simulink model "DDCU_wxt_v02_forA_LabviewV02"  (R2014a)
settings: Solver=FixedStepDiscrete  StartTime=0.0  StopTime=50  FixedStep=0.0005  RelTol=1e-3
InitFcn:
  | Veh_Par_wxt
values from neighbouring files (symbols this model uses):
  ag_thr = 0.4*g    (= 3.924)    [Veh_Par_wxt.m]
  B = 2.25    [Veh_Par_wxt.m]
  bra_pre_em = 12    [Veh_Par_wxt.m]
  bra_pre_gz2 = 12/3    (= 4)    [Veh_Par_wxt.m]
  bra_pre_gz34 = 12/3    (= 4)    [Veh_Par_wxt.m]
  bra_pre_yd = 12/2    (= 6)    [Veh_Par_wxt.m]
  brakepre_dem_data = [0 1 2 3 4 5 6 7 8 9 10 11 12]    [Veh_Par_wxt.m]
  brakeTrq_dem_data = [0 218.198 436.396 654.594 872.792 1090.99 1309.188 1527.386 1745.584 1963.782 2181.98 2400.178 2618.376]    [Veh_Par_wxt.m]
  bratrq_max = 4*2618.376    (= 10473.504)    [Veh_Par_wxt.m]
  eff_tran = 0.75    [Veh_Par_wxt.m]
  G = Mass*g    (= 36297)    [Veh_Par_wxt.m]
  kd1 = 1    [Veh_Par_wxt.m]
  kd2 = 1    [Veh_Par_wxt.m]
  kd3 = 1    [Veh_Par_wxt.m]
  ki1 = 1    [Veh_Par_wxt.m]
  ki2 = 1    [Veh_Par_wxt.m]
  ki3 = 1    [Veh_Par_wxt.m]
  kp1 = 1    [Veh_Par_wxt.m]
  kp2 = 1    [Veh_Par_wxt.m]
  kp3 = 1    [Veh_Par_wxt.m]
  L = 3.12    [Veh_Par_wxt.m]
  premax = 12    [Veh_Par_wxt.m]
  Radius = 0.20    (= 0.2)    [Veh_Par_wxt.m]
  s_opt_yi_add = 0.05    [Veh_Par_wxt.m]
  s_opt_zhuan_add = 0.05    [Veh_Par_wxt.m]
  spd_map_mot = [0 100 200 300 360 400 500 600 700 800 900]*tras_ratio    [Veh_Par_wxt.m]
  spdmax = 900*tras_ratio    (= 5580)    [Veh_Par_wxt.m]
  speed_thr_park = 5/3.6/Radius*30/pi    (= 66.3145596216)    [Veh_Par_wxt.m]
  tras_ratio = 6.2    [Veh_Par_wxt.m]
  trq_map_mot = [1200 1200 1200 1200 1200 1080 864 720 617 540 480]/tras_ratio    [Veh_Par_wxt.m]
  trqmax = 80    [Veh_Par_wxt.m]
  v_thr1_b = 5    [Veh_Par_wxt.m]
  v_thr2_b = 20    [Veh_Par_wxt.m]
  v_thr_park = 5    [Veh_Par_wxt.m]
undefined symbols (not defined in the file or in its folder): DiscIntNeverNeededParam
libraries: simulink x231, ec5744lib x19
(part 1 of 16)
settings Model: Creator=wxt  LastModifiedBy=wxt
settings OptimizationCC: InlineParams=on  InlineInvariantSignals=on  ExpressionFolding=off  RollThreshold=9  StateBitsets=on  DataBitsets=on  UseTempVars=on  ZeroExternalMemoryAtStartup=off  ZeroInternalMemoryAtStartup=off  EfficientFloat2IntCast=on  OptimizeModelRefInitCode=on  LifeSpan=1
settings DebuggingCC: InheritedTsInSrcMsg=none
settings HardwareCC: ProdLargestAtomicInteger=Long  ProdLargestAtomicFloat=Double  ProdIntDivRoundTo=Zero  ProdEndianess=BigEndian  ProdHWDeviceType=Freescale MPC5500
settings RTWCC: SystemTargetFile=ec5744.tlc  MakeCommand=make_rtw optimized_fixed_point=1  GenerateMakefile=off  TemplateMakefile=ec5744_lcc.tmf  PostCodeGenCommand=ec5744_pst_s2(buildInfo)  Description=Target for EC5744  GenerateReport=on  ProcessScript=ec5744_make_rtw_hook  IncludeHyperlinkInReport=on  LaunchReport=on
settings CodeAppCC: IgnoreCustomStorageClasses=off
settings STFCustomTargetCC: ModelReferenceCompliant=off  ConcurrentExecutionCompliant=off  IncludeMdlTerminateFcn=off  GeneratePreprocessorConditionals=Use local settings  CombineOutputUpdateFcns=on  SuppressErrorStatus=on  ERTCustomFileBanners=on  SupportContinuousTime=off  SupportNonInlinedSFcns=off  MATLABClassNameForMDSCustomization=Simulink.SoftwareTarget.ERTCustomization  GRTInterface=off  SystemTargetFile=ec5744.tlc
settings ERTTargetCC: GenerateSampleERTMain=off  ModelReferenceCompliant=off  IncludeMdlTerminateFcn=off  SuppressErrorStatus=on  GenerateASAP2=on  ERTSrcFileBannerTemplate=ec5744_code_template.cgt  ERTHdrFileBannerTemplate=ec5744_code_template.cgt  ERTDataSrcFileTemplate=ec5744_code_template.cgt  ERTDataHdrFileTemplate=ec5744_code_template.cgt  ERTCustomFileTemplate=ec5744_file_process.tlc

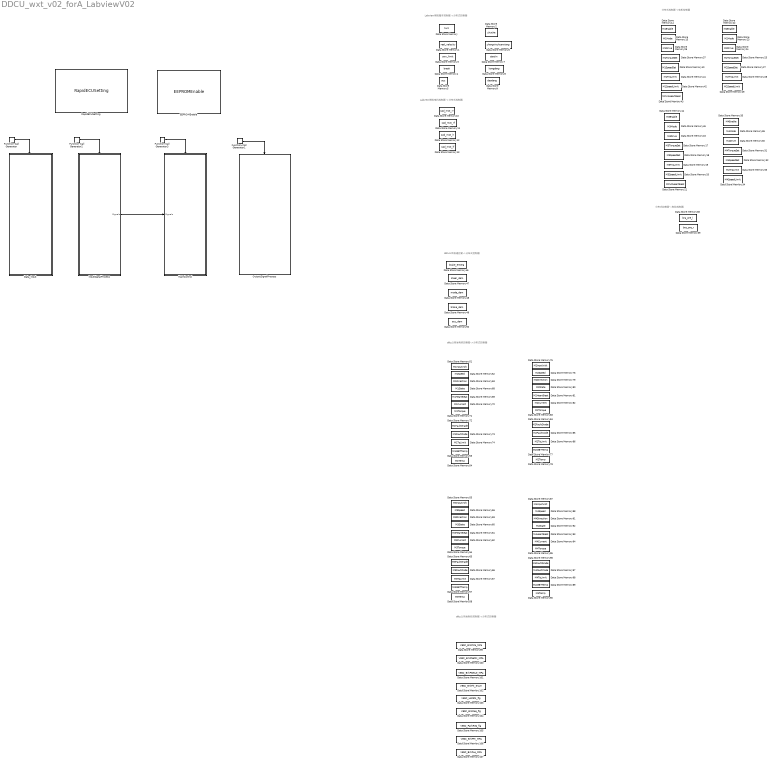
== system DDCU_wxt_v02_forA_LabviewV02 ==
  note: ddcu1转发制动控制器->分布式控制器
  note: ddcu1转发电机控制器->分布式控制器
  note: ddcu1转发遥控箱->分布式控制器
  note: Labview模拟电机控制器->分布式控制器
  note: Labview模拟整车控制器->分布式控制器
  note: 分布式控制器->制动控制器
  note: 分布式控制器->电机控制器
  Data Store Memory : DataStoreMemory  DataStoreName=turn  ReadBeforeWriteMsg=warning  WriteAfterWriteMsg=warning  WriteAfterReadMsg=warning
  Data Store Memory1 : DataStoreMemory  DataStoreName=real_velocity  ReadBeforeWriteMsg=warning  WriteAfterWriteMsg=warning  WriteAfterReadMsg=warning
  Data Store Memory10 : DataStoreMemory  DataStoreName=spd_mot_rr  ReadBeforeWriteMsg=warning  WriteAfterWriteMsg=warning  WriteAfterReadMsg=warning
  Data Store Memory100 : DataStoreMemory  DataStoreName=VESC_BrkPSetRi_MPa  ReadBeforeWriteMsg=warning  WriteAfterWriteMsg=warning  WriteAfterReadMsg=warning
  Data Store Memory101 : DataStoreMemory  DataStoreName=VESC_BrkPSetLe_MPa  ReadBeforeWriteMsg=warning  WriteAfterWriteMsg=warning  WriteAfterReadMsg=warning
  Data Store Memory102 : DataStoreMemory  DataStoreName=VESC_BrkFlt_enum  ReadBeforeWriteMsg=warning  WriteAfterWriteMsg=warning  WriteAfterReadMsg=warning
  Data Store Memory103 : DataStoreMemory  DataStoreName=VESC_HotSts_flg  ReadBeforeWriteMsg=warning  WriteAfterWriteMsg=warning  WriteAfterReadMsg=warning
  Data Store Memory104 : DataStoreMemory  DataStoreName=VESC_BrkReq_flg  ReadBeforeWriteMsg=warning  WriteAfterWriteMsg=warning  WriteAfterReadMsg=warning
  Data Store Memory105 : DataStoreMemory  DataStoreName=VESC_ParkReq_flg  ReadBeforeWriteMsg=warning  WriteAfterWriteMsg=warning  WriteAfterReadMsg=warning
  Data Store Memory106 : DataStoreMemory  DataStoreName=VESC_BrkPRi_MPa  ReadBeforeWriteMsg=warning  WriteAfterWriteMsg=warning  WriteAfterReadMsg=warning
  Data Store Memory107 : DataStoreMemory  DataStoreName=VESC_BrkPLe_MPa  ReadBeforeWriteMsg=warning  WriteAfterWriteMsg=warning  WriteAfterReadMsg=warning
  Data Store Memory11 : DataStoreMemory  DataStoreName=spd_mot_rf  ReadBeforeWriteMsg=warning  WriteAfterWriteMsg=warning  WriteAfterReadMsg=warning
  Data Store Memory12 : DataStoreMemory  DataStoreName=spd_mot_lr  ReadBeforeWriteMsg=warning  WriteAfterWriteMsg=warning  WriteAfterReadMsg=warning
  Data Store Memory13 : DataStoreMemory  DataStoreName=spd_mot_lf  ReadBeforeWriteMsg=warning  WriteAfterWriteMsg=warning  WriteAfterReadMsg=warning
  Data Store Memory14 : DataStoreMemory  DataStoreName=M1Enable  ReadBeforeWriteMsg=warning  WriteAfterWriteMsg=warning  WriteAfterReadMsg=warning
  Data Store Memory15 : DataStoreMemory  DataStoreName=M1Mode  ReadBeforeWriteMsg=warning  WriteAfterWriteMsg=warning  WriteAfterReadMsg=warning
  Data Store Memory16 : DataStoreMemory  DataStoreName=M3Drive  ReadBeforeWriteMsg=warning  WriteAfterWriteMsg=warning  WriteAfterReadMsg=warning
  Data Store Memory17 : DataStoreMemory  DataStoreName=M3TorqueSet  ReadBeforeWriteMsg=warning  WriteAfterWriteMsg=warning  WriteAfterReadMsg=warning
  Data Store Memory18 : DataStoreMemory  DataStoreName=M3SpeedSet  ReadBeforeWriteMsg=warning  WriteAfterWriteMsg=warning  WriteAfterReadMsg=warning
  Data Store Memory19 : DataStoreMemory  DataStoreName=M3TrqLimit  ReadBeforeWriteMsg=warning  WriteAfterWriteMsg=warning  WriteAfterReadMsg=warning
  Data Store Memory2 : DataStoreMemory  DataStoreName=zhuche  ReadBeforeWriteMsg=warning  WriteAfterWriteMsg=warning  WriteAfterReadMsg=warning
  Data Store Memory20 : DataStoreMemory  DataStoreName=M3SpeedLimit  ReadBeforeWriteMsg=warning  WriteAfterWriteMsg=warning  WriteAfterReadMsg=warning
  Data Store Memory21 : DataStoreMemory  DataStoreName=MCU2HeartBeat  ReadBeforeWriteMsg=warning  WriteAfterWriteMsg=warning  WriteAfterReadMsg=warning
  Data Store Memory22 : DataStoreMemory  DataStoreName=M2Enable  ReadBeforeWriteMsg=warning  WriteAfterWriteMsg=warning  WriteAfterReadMsg=warning
  Data Store Memory23 : DataStoreMemory  DataStoreName=M2Mode  ReadBeforeWriteMsg=warning  WriteAfterWriteMsg=warning  WriteAfterReadMsg=warning
  Data Store Memory24 : DataStoreMemory  DataStoreName=M2Drive  ReadBeforeWriteMsg=warning  WriteAfterWriteMsg=warning  WriteAfterReadMsg=warning
  Data Store Memory25 : DataStoreMemory  DataStoreName=M2TorqueSet  ReadBeforeWriteMsg=warning  WriteAfterWriteMsg=warning  WriteAfterReadMsg=warning
  Data Store Memory26 : DataStoreMemory  DataStoreName=M1Drive  ReadBeforeWriteMsg=warning  WriteAfterWriteMsg=warning  WriteAfterReadMsg=warning
  Data Store Memory27 : DataStoreMemory  DataStoreName=M2SpeedSet  ReadBeforeWriteMsg=warning  WriteAfterWriteMsg=warning  WriteAfterReadMsg=warning
  Data Store Memory28 : DataStoreMemory  DataStoreName=M2TrqLimit  ReadBeforeWriteMsg=warning  WriteAfterWriteMsg=warning  WriteAfterReadMsg=warning
  Data Store Memory29 : DataStoreMemory  DataStoreName=M2SpeedLimit  ReadBeforeWriteMsg=warning  WriteAfterWriteMsg=warning  WriteAfterReadMsg=warning
  Data Store Memory3 : DataStoreMemory  DataStoreName=pwr_limit  ReadBeforeWriteMsg=warning  WriteAfterWriteMsg=warning  WriteAfterReadMsg=warning
  Data Store Memory30 : DataStoreMemory  DataStoreName=M4Drive  ReadBeforeWriteMsg=warning  WriteAfterWriteMsg=warning  WriteAfterReadMsg=warning
  Data Store Memory31 : DataStoreMemory  DataStoreName=M4TorqueSet  ReadBeforeWriteMsg=warning  WriteAfterWriteMsg=warning  WriteAfterReadMsg=warning
  Data Store Memory32 : DataStoreMemory  DataStoreName=M4SpeedSet  ReadBeforeWriteMsg=warning  WriteAfterWriteMsg=warning  WriteAfterReadMsg=warning
  Data Store Memory33 : DataStoreMemory  DataStoreName=M4TrqLimit  ReadBeforeWriteMsg=warning  WriteAfterWriteMsg=warning  WriteAfterReadMsg=warning
  Data Store Memory34 : DataStoreMemory  DataStoreName=M4SpeedLimit  ReadBeforeWriteMsg=warning  WriteAfterWriteMsg=warning  WriteAfterReadMsg=warning
  Data Store Memory35 : DataStoreMemory  DataStoreName=M4Enable  ReadBeforeWriteMsg=warning  WriteAfterWriteMsg=warning  WriteAfterReadMsg=warning
  Data Store Memory36 : DataStoreMemory  DataStoreName=M4Mode  ReadBeforeWriteMsg=warning  WriteAfterWriteMsg=warning  WriteAfterReadMsg=warning
  Data Store Memory37 : DataStoreMemory  DataStoreName=M1TorqueSet  ReadBeforeWriteMsg=warning  WriteAfterWriteMsg=warning  WriteAfterReadMsg=warning
  Data Store Memory38 : DataStoreMemory  DataStoreName=bra_pre_l  ReadBeforeWriteMsg=warning  WriteAfterWriteMsg=warning  WriteAfterReadMsg=warning
  Data Store Memory39 : DataStoreMemory  DataStoreName=bra_pre_r  ReadBeforeWriteMsg=warning  WriteAfterWriteMsg=warning  WriteAfterReadMsg=warning
  Data Store Memory4 : DataStoreMemory  DataStoreName=break  ReadBeforeWriteMsg=warning  WriteAfterWriteMsg=warning  WriteAfterReadMsg=warning
  Data Store Memory40 : DataStoreMemory  DataStoreName=M1SpeedSet  ReadBeforeWriteMsg=warning  WriteAfterWriteMsg=warning  WriteAfterReadMsg=warning
  Data Store Memory41 : DataStoreMemory  DataStoreName=M1TrqLimit  ReadBeforeWriteMsg=warning  WriteAfterWriteMsg=warning  WriteAfterReadMsg=warning
  Data Store Memory42 : DataStoreMemory  DataStoreName=M1SpeedLimit  ReadBeforeWriteMsg=warning  WriteAfterWriteMsg=warning  WriteAfterReadMsg=warning
  Data Store Memory43 : DataStoreMemory  DataStoreName=MCU1HeartBeat  ReadBeforeWriteMsg=warning  WriteAfterWriteMsg=warning  WriteAfterReadMsg=warning
  Data Store Memory44 : DataStoreMemory  DataStoreName=M3Enable  ReadBeforeWriteMsg=warning  WriteAfterWriteMsg=warning  WriteAfterReadMsg=warning
  Data Store Memory45 : DataStoreMemory  DataStoreName=M3Mode  ReadBeforeWriteMsg=warning  WriteAfterWriteMsg=warning  WriteAfterReadMsg=warning
  Data Store Memory46 : DataStoreMemory  DataStoreName=brake_emerg  ReadBeforeWriteMsg=warning  WriteAfterWriteMsg=warning  WriteAfterReadMsg=warning
  Data Store Memory47 : DataStoreMemory  DataStoreName=steer_dem  ReadBeforeWriteMsg=warning  WriteAfterWriteMsg=warning  WriteAfterReadMsg=warning
  Data Store Memory48 : DataStoreMemory  DataStoreName=mode_dem  ReadBeforeWriteMsg=warning  WriteAfterWriteMsg=warning  WriteAfterReadMsg=warning
  Data Store Memory49 : DataStoreMemory  DataStoreName=brake_dem  ReadBeforeWriteMsg=warning  WriteAfterWriteMsg=warning  WriteAfterReadMsg=warning
  Data Store Memory5 : DataStoreMemory  DataStoreName=acc  ReadBeforeWriteMsg=warning  WriteAfterWriteMsg=warning  WriteAfterReadMsg=warning
  Data Store Memory50 : DataStoreMemory  DataStoreName=acc_dem  ReadBeforeWriteMsg=warning  WriteAfterWriteMsg=warning  WriteAfterReadMsg=warning
  Data Store Memory51 : DataStoreMemory  DataStoreName=M1InputVolt  ReadBeforeWriteMsg=warning  WriteAfterWriteMsg=warning  WriteAfterReadMsg=warning
  Data Store Memory52 : DataStoreMemory  DataStoreName=M1Speed  ReadBeforeWriteMsg=warning  WriteAfterWriteMsg=warning  WriteAfterReadMsg=warning
  Data Store Memory53 : DataStoreMemory  DataStoreName=M1IGBTTemp  ReadBeforeWriteMsg=warning  WriteAfterWriteMsg=warning  WriteAfterReadMsg=warning
  Data Store Memory54 : DataStoreMemory  DataStoreName=M1Temp  ReadBeforeWriteMsg=warning  WriteAfterWriteMsg=warning  WriteAfterReadMsg=warning
  Data Store Memory55 : DataStoreMemory  DataStoreName=M3InputVolt  ReadBeforeWriteMsg=warning  WriteAfterWriteMsg=warning  WriteAfterReadMsg=warning
  Data Store Memory56 : DataStoreMemory  DataStoreName=M3Speed  ReadBeforeWriteMsg=warning  WriteAfterWriteMsg=warning  WriteAfterReadMsg=warning
  Data Store Memory57 : DataStoreMemory  DataStoreName=M3IGBTTemp  ReadBeforeWriteMsg=warning  WriteAfterWriteMsg=warning  WriteAfterReadMsg=warning
  Data Store Memory58 : DataStoreMemory  DataStoreName=M3Temp  ReadBeforeWriteMsg=warning  WriteAfterWriteMsg=warning  WriteAfterReadMsg=warning
  Data Store Memory59 : DataStoreMemory  DataStoreName=M3Direction  ReadBeforeWriteMsg=warning  WriteAfterWriteMsg=warning  WriteAfterReadMsg=warning
  Data Store Memory6 : DataStoreMemory  DataStoreName=zhongxinzhuanxiang  ReadBeforeWriteMsg=warning  WriteAfterWriteMsg=warning  WriteAfterReadMsg=warning
  Data Store Memory60 : DataStoreMemory  DataStoreName=M3State  ReadBeforeWriteMsg=warning  WriteAfterWriteMsg=warning  WriteAfterReadMsg=warning
  Data Store Memory61 : DataStoreMemory  DataStoreName=M3HeartBeat  ReadBeforeWriteMsg=warning  WriteAfterWriteMsg=warning  WriteAfterReadMsg=warning
  Data Store Memory62 : DataStoreMemory  DataStoreName=M3Current  ReadBeforeWriteMsg=warning  WriteAfterWriteMsg=warning  WriteAfterReadMsg=warning
  Data Store Memory63 : DataStoreMemory  DataStoreName=M1Direction  ReadBeforeWriteMsg=warning  WriteAfterWriteMsg=warning  WriteAfterReadMsg=warning
  Data Store Memory64 : DataStoreMemory  DataStoreName=M3Torque  ReadBeforeWriteMsg=warning  WriteAfterWriteMsg=warning  WriteAfterReadMsg=warning
  Data Store Memory65 : DataStoreMemory  DataStoreName=M3FaultGrade  ReadBeforeWriteMsg=warning  WriteAfterWriteMsg=warning  WriteAfterReadMsg=warning
  Data Store Memory66 : DataStoreMemory  DataStoreName=M3FaultCode  ReadBeforeWriteMsg=warning  WriteAfterWriteMsg=warning  WriteAfterReadMsg=warning
  Data Store Memory67 : DataStoreMemory  DataStoreName=M3TqLimit  ReadBeforeWriteMsg=warning  WriteAfterWriteMsg=warning  WriteAfterReadMsg=warning
  Data Store Memory68 : DataStoreMemory  DataStoreName=M1State  ReadBeforeWriteMsg=warning  WriteAfterWriteMsg=warning  WriteAfterReadMsg=warning
  Data Store Memory69 : DataStoreMemory  DataStoreName=M1HeartBeat  ReadBeforeWriteMsg=warning  WriteAfterWriteMsg=warning  WriteAfterReadMsg=warning
  Data Store Memory7 : DataStoreMemory  DataStoreName=qianjin  ReadBeforeWriteMsg=warning  WriteAfterWriteMsg=warning  WriteAfterReadMsg=warning
  Data Store Memory70 : DataStoreMemory  DataStoreName=M1Current  ReadBeforeWriteMsg=warning  WriteAfterWriteMsg=warning  WriteAfterReadMsg=warning
  Data Store Memory71 : DataStoreMemory  DataStoreName=M1Torque  ReadBeforeWriteMsg=warning  WriteAfterWriteMsg=warning  WriteAfterReadMsg=warning
  Data Store Memory72 : DataStoreMemory  DataStoreName=M1FaultGrade  ReadBeforeWriteMsg=warning  WriteAfterWriteMsg=warning  WriteAfterReadMsg=warning
  Data Store Memory73 : DataStoreMemory  DataStoreName=M1FaultCode  ReadBeforeWriteMsg=warning  WriteAfterWriteMsg=warning  WriteAfterReadMsg=warning
  Data Store Memory74 : DataStoreMemory  DataStoreName=M1TqLimit  ReadBeforeWriteMsg=warning  WriteAfterWriteMsg=warning  WriteAfterReadMsg=warning
  Data Store Memory75 : DataStoreMemory  DataStoreName=M2InputVolt  ReadBeforeWriteMsg=warning  WriteAfterWriteMsg=warning  WriteAfterReadMsg=warning
  Data Store Memory76 : DataStoreMemory  DataStoreName=M2Speed  ReadBeforeWriteMsg=warning  WriteAfterWriteMsg=warning  WriteAfterReadMsg=warning
  Data Store Memory77 : DataStoreMemory  DataStoreName=M2IGBTTemp  ReadBeforeWriteMsg=warning  WriteAfterWriteMsg=warning  WriteAfterReadMsg=warning
  Data Store Memory78 : DataStoreMemory  DataStoreName=M2Temp  ReadBeforeWriteMsg=warning  WriteAfterWriteMsg=warning  WriteAfterReadMsg=warning
  Data Store Memory79 : DataStoreMemory  DataStoreName=M2Direction  ReadBeforeWriteMsg=warning  WriteAfterWriteMsg=warning  WriteAfterReadMsg=warning
  Data Store Memory8 : DataStoreMemory  DataStoreName=kongdang  ReadBeforeWriteMsg=warning  WriteAfterWriteMsg=warning  WriteAfterReadMsg=warning
  Data Store Memory80 : DataStoreMemory  DataStoreName=M2State  ReadBeforeWriteMsg=warning  WriteAfterWriteMsg=warning  WriteAfterReadMsg=warning
  Data Store Memory81 : DataStoreMemory  DataStoreName=M2HeartBeat  ReadBeforeWriteMsg=warning  WriteAfterWriteMsg=warning  WriteAfterReadMsg=warning
  Data Store Memory82 : DataStoreMemory  DataStoreName=M2Current  ReadBeforeWriteMsg=warning  WriteAfterWriteMsg=warning  WriteAfterReadMsg=warning
  Data Store Memory83 : DataStoreMemory  DataStoreName=M2Torque  ReadBeforeWriteMsg=warning  WriteAfterWriteMsg=warning  WriteAfterReadMsg=warning
  Data Store Memory84 : DataStoreMemory  DataStoreName=M2FaultGrade  ReadBeforeWriteMsg=warning  WriteAfterWriteMsg=warning  WriteAfterReadMsg=warning
  Data Store Memory85 : DataStoreMemory  DataStoreName=M2FaultCode  ReadBeforeWriteMsg=warning  WriteAfterWriteMsg=warning  WriteAfterReadMsg=warning
  Data Store Memory86 : DataStoreMemory  DataStoreName=M2TqLimit  ReadBeforeWriteMsg=warning  WriteAfterWriteMsg=warning  WriteAfterReadMsg=warning
  Data Store Memory87 : DataStoreMemory  DataStoreName=M4InputVolt  ReadBeforeWriteMsg=warning  WriteAfterWriteMsg=warning  WriteAfterReadMsg=warning
  Data Store Memory88 : DataStoreMemory  DataStoreName=M4Speed  ReadBeforeWriteMsg=warning  WriteAfterWriteMsg=warning  WriteAfterReadMsg=warning
  Data Store Memory89 : DataStoreMemory  DataStoreName=M4IGBTTemp  ReadBeforeWriteMsg=warning  WriteAfterWriteMsg=warning  WriteAfterReadMsg=warning
  Data Store Memory9 : DataStoreMemory  DataStoreName=daodang  ReadBeforeWriteMsg=warning  WriteAfterWriteMsg=warning  WriteAfterReadMsg=warning
  Data Store Memory90 : DataStoreMemory  DataStoreName=M4Temp  ReadBeforeWriteMsg=warning  WriteAfterWriteMsg=warning  WriteAfterReadMsg=warning
  Data Store Memory91 : DataStoreMemory  DataStoreName=M4Direction  ReadBeforeWriteMsg=warning  WriteAfterWriteMsg=warning  WriteAfterReadMsg=warning
  Data Store Memory92 : DataStoreMemory  DataStoreName=M4State  ReadBeforeWriteMsg=warning  WriteAfterWriteMsg=warning  WriteAfterReadMsg=warning
  Data Store Memory93 : DataStoreMemory  DataStoreName=M4HeartBeat  ReadBeforeWriteMsg=warning  WriteAfterWriteMsg=warning  WriteAfterReadMsg=warning
  Data Store Memory94 : DataStoreMemory  DataStoreName=M4Current  ReadBeforeWriteMsg=warning  WriteAfterWriteMsg=warning  WriteAfterReadMsg=warning
  Data Store Memory95 : DataStoreMemory  DataStoreName=M4Torque  ReadBeforeWriteMsg=warning  WriteAfterWriteMsg=warning  WriteAfterReadMsg=warning
  Data Store Memory96 : DataStoreMemory  DataStoreName=M4FaultGrade  ReadBeforeWriteMsg=warning  WriteAfterWriteMsg=warning  WriteAfterReadMsg=warning
  Data Store Memory97 : DataStoreMemory  DataStoreName=M4FaultCode  ReadBeforeWriteMsg=warning  WriteAfterWriteMsg=warning  WriteAfterReadMsg=warning
  Data Store Memory98 : DataStoreMemory  DataStoreName=M4TqLimit  ReadBeforeWriteMsg=warning  WriteAfterWriteMsg=warning  WriteAfterReadMsg=warning
  Data Store Memory99 : DataStoreMemory  DataStoreName=VESC_BrkPMa_MPa  ReadBeforeWriteMsg=warning  WriteAfterWriteMsg=warning  WriteAfterReadMsg=warning
  Data_Input : Subsystem  TreatAsAtomicUnit=on
  EEPROMEnable : ec5744lib/RapidECU_U3/09MemoryManagement/EEPROMEnable  eepromenable=on
  Function-Call Generator{,1..3} (4 alike) : simulink/Ports & Subsystems/Function-Call Generator  sample_time=0.05  numberOfIterations=1
  InputSignalProcess : Subsystem
  MainControl : Subsystem
  OutputSignalProcess : Subsystem  TreatAsAtomicUnit=on
  RapidECUSetting : ec5744lib/RapidECU_U3/RapidECUSetting
      link override CAN: apdf=4  bpdf=4  cpdf=4  acmt=Extended(29-bit ID)  bcmt=Extended(29-bit ID)
      link override LIN: abrt=19200
  wires:
  Function-Call Generator/1 -> Data_Input/Trigger
  Function-Call Generator1/1 -> OutputSignalProcess/Trigger
  Function-Call Generator2/1 -> InputSignalProcess/Trigger
  InputSignalProcess/1(Signals) -> MainControl/1(Signals)
  Function-Call Generator3/1 -> MainControl/Trigger

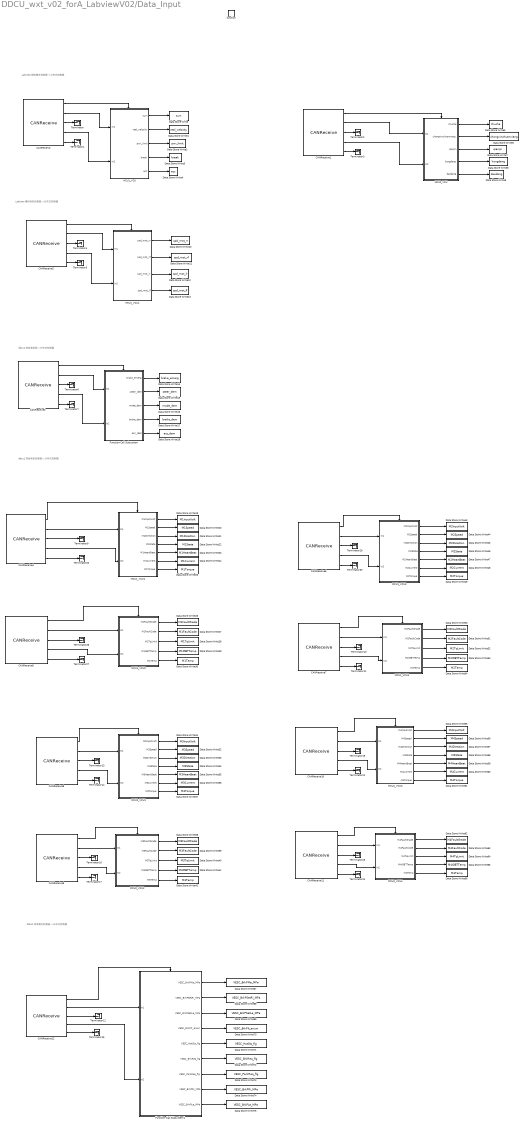
== system DDCU_wxt_v02_forA_LabviewV02/Data_Input ==
  note: ddcu1转发制动控制器->分布式控制器
  note: ddcu1转发电机控制器->分布式控制器
  note: ddcu1转发遥控箱->分布式控制器
  note: Labview模拟电机控制器->分布式控制器
  note: Labview模拟整车控制器->分布式控制器
  function : TriggerPort  TriggerType=function-call
  CANReceive : ec5744lib/RapidECU_U3/04CANCommunication/CANReceive  canmodule=0  canbuffer=0  canmessageid=hex2dec('1502C23A')  canmessagetype=Extended(29-bit ID)  datalength=8  sampletime=-1
  CANReceive1 : ec5744lib/RapidECU_U3/04CANCommunication/CANReceive  canmodule=0  canbuffer=1  canmessageid=hex2dec('0902C23A')  canmessagetype=Extended(29-bit ID)  datalength=8  sampletime=-1
  CANReceive10 : ec5744lib/RapidECU_U3/04CANCommunication/CANReceive  canmodule=0  canbuffer=16  canmessageid=hex2dec('0C0302F0')  canmessagetype=Extended(29-bit ID)  datalength=8  sampletime=-1
  CANReceive11 : ec5744lib/RapidECU_U3/04CANCommunication/CANReceive  canmodule=0  canbuffer=17  canmessageid=hex2dec('0C0402F0')  canmessagetype=Extended(29-bit ID)  datalength=8  sampletime=-1
  CANReceive12 : ec5744lib/RapidECU_U3/04CANCommunication/CANReceive  canmodule=1  canbuffer=20  canmessageid=hex2dec('0CF6F0EA')  canmessagetype=Extended(29-bit ID)  datalength=8  sampletime=-1
  CANReceive2 : ec5744lib/RapidECU_U3/04CANCommunication/CANReceive  canmodule=0  canbuffer=2  canmessageid=hex2dec('0C0101F0')  canmessagetype=Extended(29-bit ID)  datalength=8  sampletime=-1
  CANReceive3 : ec5744lib/RapidECU_U3/04CANCommunication/CANReceive  canmodule=0  canbuffer=0  canmessageid=hex2dec('1502C23A')  canmessagetype=Extended(29-bit ID)  datalength=8  sampletime=-1
  CANReceive4 : ec5744lib/RapidECU_U3/04CANCommunication/CANReceive  canmodule=0  canbuffer=2  canmessageid=hex2dec('0C0101F0')  canmessagetype=Extended(29-bit ID)  datalength=8  sampletime=-1
  CANReceive5 : ec5744lib/RapidECU_U3/04CANCommunication/CANReceive  canmodule=0  canbuffer=3  canmessageid=hex2dec('0C0201F0')  canmessagetype=Extended(29-bit ID)  datalength=8  sampletime=-1
  CANReceive6 : ec5744lib/RapidECU_U3/04CANCommunication/CANReceive  canmodule=0  canbuffer=4  canmessageid=hex2dec('0C0301F0')  canmessagetype=Extended(29-bit ID)  datalength=8  sampletime=-1
  CANReceive7 : ec5744lib/RapidECU_U3/04CANCommunication/CANReceive  canmodule=0  canbuffer=5  canmessageid=hex2dec('0C0401F0')  canmessagetype=Extended(29-bit ID)  datalength=8  sampletime=-1
  CANReceive8 : ec5744lib/RapidECU_U3/04CANCommunication/CANReceive  canmodule=0  canbuffer=6  canmessageid=hex2dec('0C0102F0')  canmessagetype=Extended(29-bit ID)  datalength=8  sampletime=-1
  CANReceive9 : ec5744lib/RapidECU_U3/04CANCommunication/CANReceive  canmodule=0  canbuffer=7  canmessageid=hex2dec('0C0202F0')  canmessagetype=Extended(29-bit ID)  datalength=8  sampletime=-1
  Data Store Write : DataStoreWrite  DialogController=Simulink.DDGSource  DataStoreName=turn  DataStoreElements=turn
  Data Store Write1 : DataStoreWrite  DataStoreName=real_velocity
  Data Store Write10 : DataStoreWrite  DataStoreName=spd_mot_rr
  Data Store Write11 : DataStoreWrite  DataStoreName=spd_mot_rf
  Data Store Write12 : DataStoreWrite  DataStoreName=spd_mot_lr
  Data Store Write13 : DataStoreWrite  DialogController=Simulink.DDGSource  DataStoreName=spd_mot_lf  DataStoreElements=spd_mot_lf
  Data Store Write14 : DataStoreWrite  DialogController=Simulink.DDGSource  DataStoreName=brake_emerg
  Data Store Write15 : DataStoreWrite  DataStoreName=steer_dem
  Data Store Write16 : DataStoreWrite  DataStoreName=mode_dem
  Data Store Write17 : DataStoreWrite  DataStoreName=brake_dem
  Data Store Write18 : DataStoreWrite  DataStoreName=acc_dem
  Data Store Write19 : DataStoreWrite  DataStoreName=M1InputVolt
  Data Store Write2 : DataStoreWrite  DataStoreName=pwr_limit
  Data Store Write20 : DataStoreWrite  DataStoreName=M1Speed
  Data Store Write21 : DataStoreWrite  DataStoreName=M1Direction
  Data Store Write22 : DataStoreWrite  DataStoreName=M1State
  Data Store Write23 : DataStoreWrite  DataStoreName=M1HeartBeat
  Data Store Write24 : DataStoreWrite  DataStoreName=M1Current
  Data Store Write25 : DataStoreWrite  DataStoreName=M1Torque
  Data Store Write26 : DataStoreWrite  DataStoreName=M1FaultGrade
  Data Store Write27 : DataStoreWrite  DataStoreName=M1FaultCode
  Data Store Write28 : DataStoreWrite  DialogController=Simulink.DDGSource  DataStoreName=M1TqLimit
  Data Store Write29 : DataStoreWrite  DataStoreName=M1IGBTTemp
  Data Store Write3 : DataStoreWrite  DataStoreName=break
  Data Store Write30 : DataStoreWrite  DataStoreName=M1Temp
  Data Store Write31 : DataStoreWrite  DataStoreName=M3InputVolt
  Data Store Write32 : DataStoreWrite  DataStoreName=M3Speed
  Data Store Write33 : DataStoreWrite  DataStoreName=M3Direction
  Data Store Write34 : DataStoreWrite  DataStoreName=M3State
  Data Store Write35 : DataStoreWrite  DataStoreName=M3HeartBeat
  Data Store Write36 : DataStoreWrite  DataStoreName=M3Current
  Data Store Write37 : DataStoreWrite  DataStoreName=M3Torque
  Data Store Write38 : DataStoreWrite  DataStoreName=M3FaultGrade
  Data Store Write39 : DataStoreWrite  DataStoreName=M3FaultCode
  Data Store Write4 : DataStoreWrite  DataStoreName=acc
  Data Store Write40 : DataStoreWrite  DataStoreName=M3TqLimit
  Data Store Write41 : DataStoreWrite  DataStoreName=M3IGBTTemp
  Data Store Write42 : DataStoreWrite  DataStoreName=M3Temp
  Data Store Write43 : DataStoreWrite  DataStoreName=M2InputVolt
  Data Store Write44 : DataStoreWrite  DataStoreName=M2Speed
  Data Store Write45 : DataStoreWrite  DataStoreName=M2Direction
  Data Store Write46 : DataStoreWrite  DataStoreName=M2State
  Data Store Write47 : DataStoreWrite  DataStoreName=M2HeartBeat
  Data Store Write48 : DataStoreWrite  DataStoreName=M2Current
  Data Store Write49 : DataStoreWrite  DataStoreName=M2Torque
  Data Store Write5 : DataStoreWrite  DataStoreName=zhuche
  Data Store Write50 : DataStoreWrite  DataStoreName=M2FaultGrade
  Data Store Write51 : DataStoreWrite  DataStoreName=M2FaultCode
  Data Store Write52 : DataStoreWrite  DataStoreName=M2TqLimit
  Data Store Write53 : DataStoreWrite  DataStoreName=M2IGBTTemp
  Data Store Write54 : DataStoreWrite  DataStoreName=M2Temp
  Data Store Write55 : DataStoreWrite  DataStoreName=M4InputVolt
  Data Store Write56 : DataStoreWrite  DataStoreName=M4Speed
  Data Store Write57 : DataStoreWrite  DataStoreName=M4Direction
  Data Store Write58 : DataStoreWrite  DataStoreName=M4State
  Data Store Write59 : DataStoreWrite  DataStoreName=M4HeartBeat
  Data Store Write6 : DataStoreWrite  DataStoreName=zhongxinzhuanxiang
  Data Store Write60 : DataStoreWrite  DataStoreName=M4Current
  Data Store Write61 : DataStoreWrite  DataStoreName=M4Torque
  Data Store Write62 : DataStoreWrite  DataStoreName=M4FaultGrade
  Data Store Write63 : DataStoreWrite  DataStoreName=M4FaultCode
  Data Store Write64 : DataStoreWrite  DataStoreName=M4TqLimit
  Data Store Write65 : DataStoreWrite  DataStoreName=M4IGBTTemp
  Data Store Write66 : DataStoreWrite  DataStoreName=M4Temp
  Data Store Write67 : DataStoreWrite  DataStoreName=VESC_BrkPMa_MPa
  Data Store Write68 : DataStoreWrite  DataStoreName=VESC_BrkPSetRi_MPa
  Data Store Write69 : DataStoreWrite  DataStoreName=VESC_BrkPSetLe_MPa
  Data Store Write7 : DataStoreWrite  DataStoreName=qianjin
  Data Store Write70 : DataStoreWrite  DataStoreName=VESC_BrkFlt_enum
  Data Store Write71 : DataStoreWrite  DataStoreName=VESC_HotSts_flg
  Data Store Write72 : DataStoreWrite  DataStoreName=VESC_BrkReq_flg
  Data Store Write73 : DataStoreWrite  DataStoreName=VESC_ParkReq_flg
  Data Store Write74 : DataStoreWrite  DataStoreName=VESC_BrkPRi_MPa
  Data Store Write75 : DataStoreWrite  DataStoreName=VESC_BrkPLe_MPa
  Data Store Write8 : DataStoreWrite  DataStoreName=kongdang
  Data Store Write9 : DataStoreWrite  DataStoreName=daodang
  Function-Call Subsystem : Subsystem  TreatAsAtomicUnit=on
  Function-Call Subsystem1 : Subsystem  TreatAsAtomicUnit=on
  HCU1_VCU : Subsystem  TreatAsAtomicUnit=on
  HCU1_VCU1 : Subsystem  TreatAsAtomicUnit=on
  HCU2_VCU : Subsystem  TreatAsAtomicUnit=on
  MCU1_VCU1 : Subsystem  TreatAsAtomicUnit=on
  MCU1_VCU2 : Subsystem  TreatAsAtomicUnit=on
  MCU1_VCU3 : Subsystem  TreatAsAtomicUnit=on
  MCU1_VCU4 : Subsystem  TreatAsAtomicUnit=on
  MCU2_VCU1 : Subsystem  TreatAsAtomicUnit=on
  MCU2_VCU2 : Subsystem  TreatAsAtomicUnit=on
  MCU2_VCU3 : Subsystem  TreatAsAtomicUnit=on
  MCU2_VCU4 : Subsystem  TreatAsAtomicUnit=on
  Terminator{,1..7,9..17,19..21,23..24,26..27,29..30} (26 alike) : Terminator
  wires:
  CANReceive/1 -> HCU1_VCU/Trigger
  CANReceive/2 -> HCU1_VCU/1(In1)
  CANReceive/4 -> HCU1_VCU/2(In2)
  CANReceive/3 -> Terminator/1
  CANReceive/5 -> Terminator1/1
  HCU1_VCU/3(pwr_limit) -> Data Store Write2/1
  HCU1_VCU/2(real_velocity) -> Data Store Write1/1
  HCU1_VCU/4(break) -> Data Store Write3/1
  HCU1_VCU/1(turn) -> Data Store Write/1
  HCU1_VCU/5(acc) -> Data Store Write4/1
  CANReceive1/1 -> HCU2_VCU/Trigger
  CANReceive1/2 -> HCU2_VCU/1(In1)
  CANReceive1/4 -> HCU2_VCU/2(In2)
  CANReceive1/3 -> Terminator2/1
  CANReceive1/5 -> Terminator3/1
  HCU2_VCU/3(qianjin) -> Data Store Write7/1
  HCU2_VCU/4(kongdang) -> Data Store Write8/1
  HCU2_VCU/2(zhongxinzhuanxiang) -> Data Store Write6/1
  HCU2_VCU/1(zhuche) -> Data Store Write5/1
  HCU2_VCU/5(daodang) -> Data Store Write9/1
  CANReceive2/1 -> HCU1_VCU1/Trigger
  CANReceive2/2 -> HCU1_VCU1/1(In1)
  CANReceive2/4 -> HCU1_VCU1/2(In2)
  CANReceive2/3 -> Terminator4/1
  CANReceive2/5 -> Terminator5/1
  HCU1_VCU1/1(spd_mot_rr) -> Data Store Write10/1
  HCU1_VCU1/2(spd_mot_rf) -> Data Store Write11/1
  HCU1_VCU1/3(spd_mot_lr) -> Data Store Write12/1
  HCU1_VCU1/4(spd_mot_lf) -> Data Store Write13/1
  Function-Call Subsystem/1(brake_emerg) -> Data Store Write14/1
  Function-Call Subsystem/2(steer_dem) -> Data Store Write15/1
  Function-Call Subsystem/3(mode_dem) -> Data Store Write16/1
  Function-Call Subsystem/4(brake_dem) -> Data Store Write17/1
  Function-Call Subsystem/5(acc_dem) -> Data Store Write18/1
  CANReceive3/1 -> Function-Call Subsystem/Trigger
  CANReceive3/2 -> Function-Call Subsystem/1(In1)
  CANReceive3/4 -> Function-Call Subsystem/2(In2)
  CANReceive3/3 -> Terminator6/1
  CANReceive3/5 -> Terminator7/1
  CANReceive4/4 -> MCU1_VCU1/2(In2)
  CANReceive4/2 -> MCU1_VCU1/1(In1)
  CANReceive4/3 -> Terminator9/1
  CANReceive4/5 -> Terminator20/1
  CANReceive5/4 -> MCU1_VCU2/2(In2)
  CANReceive5/2 -> MCU1_VCU2/1(In1)
  CANReceive5/3 -> Terminator26/1
  CANReceive5/5 -> Terminator27/1
  CANReceive6/4 -> MCU1_VCU3/2(In2)
  CANReceive7/4 -> MCU1_VCU4/2(In2)
  CANReceive6/5 -> Terminator30/1
  CANReceive6/2 -> MCU1_VCU3/1(In1)
  CANReceive6/3 -> Terminator29/1
  CANReceive7/3 -> Terminator10/1
  CANReceive7/5 -> Terminator11/1
  CANReceive7/2 -> MCU1_VCU4/1(In1)
  CANReceive8/4 -> MCU2_VCU1/2(In2)
  CANReceive8/2 -> MCU2_VCU1/1(In1)
  CANReceive8/3 -> Terminator13/1
  CANReceive8/5 -> Terminator14/1
  CANReceive9/4 -> MCU2_VCU2/2(In2)
  CANReceive9/2 -> MCU2_VCU2/1(In1)
  CANReceive9/3 -> Terminator16/1
  CANReceive9/5 -> Terminator17/1
  CANReceive10/4 -> MCU2_VCU3/2(In2)
  CANReceive10/2 -> MCU2_VCU3/1(In1)
  CANReceive10/3 -> Terminator19/1
  CANReceive10/5 -> Terminator21/1
  CANReceive11/4 -> MCU2_VCU4/2(In2)
  CANReceive11/2 -> MCU2_VCU4/1(In1)
  CANReceive11/3 -> Terminator23/1
  CANReceive11/5 -> Terminator24/1
  CANReceive5/1 -> MCU1_VCU2/Trigger
  CANReceive6/1 -> MCU1_VCU3/Trigger
  CANReceive7/1 -> MCU1_VCU4/Trigger
  CANReceive8/1 -> MCU2_VCU1/Trigger
  CANReceive9/1 -> MCU2_VCU2/Trigger
  CANReceive10/1 -> MCU2_VCU3/Trigger
  CANReceive11/1 -> MCU2_VCU4/Trigger
  CANReceive4/1 -> MCU1_VCU1/Trigger
  CANReceive12/5 -> Terminator15/1
  CANReceive12/2 -> Function-Call Subsystem1/1(In1)
  CANReceive12/3 -> Terminator12/1
  CANReceive12/1 -> Function-Call Subsystem1/Trigger
  CANReceive12/4 -> Function-Call Subsystem1/2(In2)
  MCU1_VCU1/2(M1Speed) -> Data Store Write20/1
  MCU1_VCU1/4(M1State) -> Data Store Write22/1
  MCU1_VCU1/3(M1Direction) -> Data Store Write21/1
  MCU1_VCU1/1(M1InputVolt) -> Data Store Write19/1
  MCU1_VCU1/5(M1HeartBeat) -> Data Store Write23/1
  MCU1_VCU1/6(M1Current) -> Data Store Write24/1
  MCU1_VCU1/7(M1Torque) -> Data Store Write25/1
  MCU1_VCU2/1(M1FaultGrade) -> Data Store Write26/1
  MCU1_VCU2/2(M1FaultCode) -> Data Store Write27/1
  MCU1_VCU2/3(M1TqLimit) -> Data Store Write28/1
  MCU1_VCU2/4(M1IGBTTemp) -> Data Store Write29/1
  MCU1_VCU2/5(M1Temp) -> Data Store Write30/1
  MCU2_VCU3/1(M4InputVolt) -> Data Store Write55/1
  MCU2_VCU3/4(M4State) -> Data Store Write58/1
  MCU2_VCU3/3(M4Direction) -> Data Store Write57/1
  MCU2_VCU3/2(M4Speed) -> Data Store Write56/1
  MCU2_VCU3/5(M4HeartBeat) -> Data Store Write59/1
  MCU2_VCU3/6(M4Current) -> Data Store Write60/1
  MCU2_VCU3/7(M4Torque) -> Data Store Write61/1
  MCU2_VCU1/4(M3State) -> Data Store Write34/1
  MCU2_VCU1/1(M3InputVolt) -> Data Store Write31/1
  MCU2_VCU1/5(M3HeartBeat) -> Data Store Write35/1
  MCU2_VCU1/2(M3Speed) -> Data Store Write32/1
  MCU2_VCU1/3(M3Direction) -> Data Store Write33/1
  MCU2_VCU1/6(M3Current) -> Data Store Write36/1
  MCU2_VCU1/7(M3Torque) -> Data Store Write37/1
  MCU2_VCU2/2(M3FaultCode) -> Data Store Write39/1
  MCU2_VCU2/1(M3FaultGrade) -> Data Store Write38/1
  MCU2_VCU2/5(M3Temp) -> Data Store Write42/1
  MCU2_VCU2/4(M3IGBTTemp) -> Data Store Write41/1
  MCU2_VCU2/3(M3TqLimit) -> Data Store Write40/1
  MCU1_VCU3/1(M2InputVolt) -> Data Store Write43/1
  MCU1_VCU3/2(M2Speed) -> Data Store Write44/1
  MCU1_VCU3/3(M2Direction) -> Data Store Write45/1
  MCU1_VCU3/4(M2State) -> Data Store Write46/1
  MCU1_VCU3/5(M2HeartBeat) -> Data Store Write47/1
  MCU1_VCU3/6(M2Current) -> Data Store Write48/1
  MCU1_VCU3/7(M2Torque) -> Data Store Write49/1
  MCU1_VCU4/4(M2IGBTTemp) -> Data Store Write53/1
  MCU1_VCU4/5(M2Temp) -> Data Store Write54/1
  MCU1_VCU4/2(M2FaultCode) -> Data Store Write51/1
  MCU1_VCU4/1(M2FaultGrade) -> Data Store Write50/1
  MCU1_VCU4/3(M2TqLimit) -> Data Store Write52/1
  MCU2_VCU4/5(M4Temp) -> Data Store Write66/1
  MCU2_VCU4/4(M4IGBTTemp) -> Data Store Write65/1
  MCU2_VCU4/3(M4TqLimit) -> Data Store Write64/1
  MCU2_VCU4/2(M4FaultCode) -> Data Store Write63/1
  MCU2_VCU4/1(M4FaultGrade) -> Data Store Write62/1
  Function-Call Subsystem1/1(VESC_BrkPMa_MPa) -> Data Store Write67/1
  Function-Call Subsystem1/2(VESC_BrkPSetRi_MPa) -> Data Store Write68/1
  Function-Call Subsystem1/4(VESC_BrkFlt_enum) -> Data Store Write70/1
  Function-Call Subsystem1/3(VESC_BrkPSetLe_MPa) -> Data Store Write69/1
  Function-Call Subsystem1/6(VESC_BrkReq_flg) -> Data Store Write72/1
  Function-Call Subsystem1/5(VESC_HotSts_flg) -> Data Store Write71/1
  Function-Call Subsystem1/7(VESC_ParkReq_flg) -> Data Store Write73/1
  Function-Call Subsystem1/8(VESC_BrkPRi_MPa) -> Data Store Write74/1
  Function-Call Subsystem1/9(VESC_BrkPLe_MPa) -> Data Store Write75/1

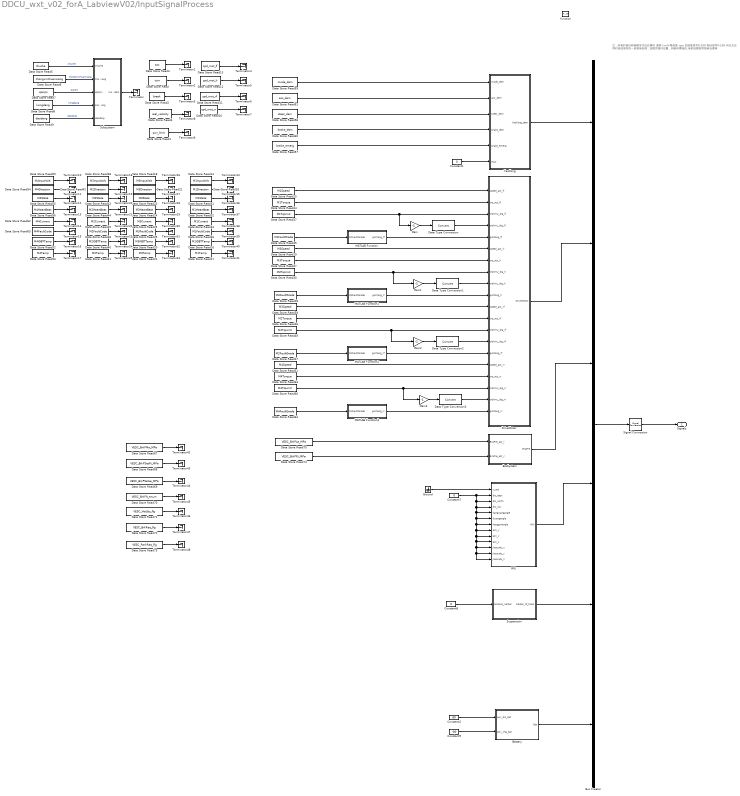
== system DDCU_wxt_v02_forA_LabviewV02/InputSignalProcess ==
  note: 注：所有的单位转换都发生在此模块
      | 速度 km/h
      | 角速度 rpm
      | 加速度信号0-100
      | 制动信号0-100
      | 向左为正
      | 同时包括信号的一些简单处理，如根究摇杆位置，判断所需档位,电机故障信号简单处理等
  function : TriggerPort  TriggerType=function-call
  Battery : Subsystem
  BraSystem : Subsystem
  Bus Creator : BusCreator  Inputs=6
  Constant1 : Constant  Value=0
  Constant2 : Constant  Value=80
  Constant7 : Constant  Value=0
  Constant8 : Constant  Value=0
  Constant9 : Constant  Value=-80
  Data Store Read : DataStoreRead  DialogController=Simulink.DDGSource  DataStoreName=turn  DataStoreElements=turn
  Data Store Read1 : DataStoreRead  DataStoreName=pwr_limit
  Data Store Read10 : DataStoreRead  DataStoreName=spd_mot_rr
  Data Store Read11 : DataStoreRead  DataStoreName=spd_mot_rf
  Data Store Read12 : DataStoreRead  DataStoreName=spd_mot_lr
  Data Store Read13 : DataStoreRead  DataStoreName=spd_mot_lf  DataStoreElements=spd_mot_lf
  Data Store Read14 : DataStoreRead  DataStoreName=M1InputVolt
  Data Store Read15 : DataStoreRead  DataStoreName=M1Speed
  Data Store Read16 : DataStoreRead  DataStoreName=M1IGBTTemp
  Data Store Read17 : DataStoreRead  DataStoreName=M1Temp
  Data Store Read18 : DataStoreRead  DataStoreName=M3InputVolt
  Data Store Read19 : DataStoreRead  DataStoreName=M3Speed
  Data Store Read2 : DataStoreRead  DataStoreName=break
  Data Store Read20 : DataStoreRead  DataStoreName=M3IGBTTemp
  Data Store Read21 : DataStoreRead  DataStoreName=M3Temp
  Data Store Read22 : DataStoreRead  DataStoreName=M3Direction
  Data Store Read23 : DataStoreRead  DataStoreName=M3State
  Data Store Read24 : DataStoreRead  DataStoreName=M3HeartBeat
  Data Store Read25 : DataStoreRead  DataStoreName=M3Current
  Data Store Read26 : DataStoreRead  DataStoreName=M1Direction
  Data Store Read27 : DataStoreRead  DataStoreName=M3Torque
  Data Store Read28 : DataStoreRead  DataStoreName=M3FaultGrade
  Data Store Read29 : DataStoreRead  DataStoreName=M3FaultCode
  Data Store Read3 : DataStoreRead  DataStoreName=acc
  Data Store Read30 : DataStoreRead  DataStoreName=M3TqLimit
  Data Store Read31 : DataStoreRead  DataStoreName=M1State
  Data Store Read32 : DataStoreRead  DataStoreName=M1HeartBeat
  Data Store Read33 : DataStoreRead  DataStoreName=M1Current
  Data Store Read34 : DataStoreRead  DataStoreName=M1Torque
  Data Store Read35 : DataStoreRead  DataStoreName=M1FaultGrade
  Data Store Read36 : DataStoreRead  DataStoreName=M1FaultCode
  Data Store Read37 : DataStoreRead  DataStoreName=M1TqLimit
  Data Store Read38 : DataStoreRead  DataStoreName=M2InputVolt
  Data Store Read39 : DataStoreRead  DataStoreName=M2Speed
  Data Store Read4 : DataStoreRead  DataStoreName=real_velocity
  Data Store Read40 : DataStoreRead  DataStoreName=M2IGBTTemp
  Data Store Read41 : DataStoreRead  DataStoreName=M2Temp
  Data Store Read42 : DataStoreRead  DataStoreName=M2Direction
  Data Store Read43 : DataStoreRead  DataStoreName=M2State
  Data Store Read44 : DataStoreRead  DataStoreName=M2HeartBeat
  Data Store Read45 : DataStoreRead  DataStoreName=M2Current
  Data Store Read46 : DataStoreRead  DataStoreName=M2Torque
  Data Store Read47 : DataStoreRead  DataStoreName=M2FaultGrade
  Data Store Read48 : DataStoreRead  DataStoreName=M2FaultCode
  Data Store Read49 : DataStoreRead  DataStoreName=M2TqLimit
  Data Store Read5 : DataStoreRead  DataStoreName=zhuche
  Data Store Read50 : DataStoreRead  DataStoreName=M4InputVolt
  Data Store Read51 : DataStoreRead  DataStoreName=M4Speed
  Data Store Read52 : DataStoreRead  DataStoreName=M4IGBTTemp
  Data Store Read53 : DataStoreRead  DataStoreName=M4Temp
  Data Store Read54 : DataStoreRead  DataStoreName=M4Direction
  Data Store Read55 : DataStoreRead  DataStoreName=M4State
  Data Store Read56 : DataStoreRead  DataStoreName=M4HeartBeat
  Data Store Read57 : DataStoreRead  DataStoreName=brake_emerg
  Data Store Read58 : DataStoreRead  DataStoreName=steer_dem
  Data Store Read59 : DataStoreRead  DataStoreName=mode_dem
  Data Store Read6 : DataStoreRead  DataStoreName=zhongxinzhuanxiang
  Data Store Read60 : DataStoreRead  DataStoreName=brake_dem
  Data Store Read61 : DataStoreRead  DataStoreName=acc_dem
  Data Store Read62 : DataStoreRead  DataStoreName=M4Current
  Data Store Read63 : DataStoreRead  DataStoreName=M4Torque
  Data Store Read64 : DataStoreRead  DataStoreName=M4FaultGrade
  Data Store Read65 : DataStoreRead  DataStoreName=M4FaultCode
  Data Store Read66 : DataStoreRead  DataStoreName=M4TqLimit
  Data Store Read67 : DataStoreRead  DataStoreName=VESC_BrkPMa_MPa
  Data Store Read68 : DataStoreRead  DataStoreName=VESC_BrkPSetRi_MPa
  Data Store Read69 : DataStoreRead  DataStoreName=VESC_BrkPSetLe_MPa
  Data Store Read7 : DataStoreRead  DataStoreName=qianjin
  Data Store Read70 : DataStoreRead  DataStoreName=VESC_BrkFlt_enum
  Data Store Read71 : DataStoreRead  DataStoreName=VESC_HotSts_flg
  Data Store Read72 : DataStoreRead  DataStoreName=VESC_BrkReq_flg
  Data Store Read73 : DataStoreRead  DataStoreName=VESC_ParkReq_flg
  Data Store Read74 : DataStoreRead  DataStoreName=VESC_BrkPRi_MPa
  Data Store Read75 : DataStoreRead  DataStoreName=VESC_BrkPLe_MPa
  Data Store Read8 : DataStoreRead  DataStoreName=kongdang
  Data Store Read9 : DataStoreRead  DataStoreName=daodang
  Data Type Conversion{,1..3} (4 alike) : DataTypeConversion
  DriveMotor : Subsystem
  Gain{,1..3} (4 alike) : Gain  Gain=-1
  Ground : Ground
  IMU : Subsystem
  MATLAB Function : MATLAB Function  TreatAsAtomicUnit=on
  MATLAB Function1 : MATLAB Function  TreatAsAtomicUnit=on
  MATLAB Function2 : MATLAB Function  TreatAsAtomicUnit=on
  MATLAB Function3 : MATLAB Function  TreatAsAtomicUnit=on
  Signal Conversion : SignalConversion
  Subsystem : Subsystem
  Suspension : Subsystem
  Terminator{,1..48} (49 alike) : Terminator
  YaoKong : Subsystem
  Signals : Outport
  wires:
  DriveMotor/1(DriveMotor) -> Bus Creator/2
  BraSystem/1(BraPre) -> Bus Creator/3
  YaoKong/1(YaoKong_dem) -> Bus Creator/1
  IMU/1(IMU) -> Bus Creator/4
  Suspension/1(Center_of_Mass) -> Bus Creator/5
  Battery/1(Bat) -> Bus Creator/6
  Constant8/1 -> Suspension/1(location_center)
  Constant9/1 -> Battery/2(pwr_chg_bat)
  Data Store Read6/1 -> Subsystem/2(zhongxinzhuanxiang)  "zhongxinzhuanxiang"
  Data Store Read7/1 -> Subsystem/3(qianjin)  "qianjin"
  Data Store Read8/1 -> Subsystem/4(kongdang)  "kongdang"
  Data Store Read9/1 -> Subsystem/5(daodang)  "daodang"
  Data Store Read61/1 -> YaoKong/2(acc_dem)
  Data Store Read58/1 -> YaoKong/3(steer_dem)
  Ground/1 -> IMU/1(v_act)
  Data Store Read51/1 -> DriveMotor/16(speed_act_rr)
  Data Store Read39/1 -> DriveMotor/11(speed_act_rf)
  Data Store Read19/1 -> DriveMotor/6(speed_act_lr)
  Data Store Read15/1 -> DriveMotor/1(speed_act_lf)
  Bus Creator/1 -> Signal Conversion/1
  Data Store Read57/1 -> YaoKong/5(brake_emerg)
  Constant1/1 -> YaoKong/6(HAC)
  Constant7/1 -> IMU/3(dis_north), IMU/4(dis_sky), IMU/5(hangxiangangle), IMU/6(fuyangangle), IMU/7(henggunangle), IMU/8(acc_x), IMU/9(acc_y), IMU/10(acc_z), IMU/11(jiaosudu_x), IMU/12(jiaosudu_y), IMU/13(jiaosudu_z), IMU/2(dis_east)
  Data Store Read5/1 -> Subsystem/1(zhuche)  "zhuche"
  Signal Conversion/1 -> Signals/1
  Data Store Read35/1 -> MATLAB Function/1(M1FaultGrade)
  Data Store Read37/1 -> Gain/1, DriveMotor/3(trqlimU_dig_lf)
  Gain/1 -> Data Type Conversion/1
  Data Store Read28/1 -> MATLAB Function1/1(M3FaultGrade)
  Data Store Read30/1 -> Gain1/1, DriveMotor/8(trqlimU_dig_lr)
  Gain1/1 -> Data Type Conversion1/1
  Data Store Read47/1 -> MATLAB Function2/1(M2FaultGrade)
  Gain2/1 -> Data Type Conversion2/1
  Data Store Read64/1 -> MATLAB Function3/1(M4FaultGrade)
  Data Store Read66/1 -> Gain3/1, DriveMotor/18(trqlimU_dig_rr)
  Subsystem/1(mode_dem) -> Terminator/1
  Data Store Read3/1 -> Terminator1/1
  Data Store Read/1 -> Terminator2/1
  Data Store Read2/1 -> Terminator3/1
  Data Store Read13/1 -> Terminator4/1
  Data Store Read12/1 -> Terminator5/1
  Data Store Read11/1 -> Terminator6/1
  Data Store Read10/1 -> Terminator7/1
  Data Store Read59/1 -> YaoKong/1(mode_dem)
  Data Store Read60/1 -> YaoKong/4(brake_dem)
  Data Store Read4/1 -> Terminator8/1
  Data Store Read1/1 -> Terminator9/1
  Data Store Read34/1 -> DriveMotor/2(trq_act_lf)
  Data Store Read27/1 -> DriveMotor/7(trq_act_lr)
  Data Store Read46/1 -> DriveMotor/12(trq_act_rf)
  Data Store Read49/1 -> Gain2/1, DriveMotor/13(trqlimU_dig_rf)
  Data Store Read63/1 -> DriveMotor/17(trq_act_rr)
  Gain3/1 -> Data Type Conversion3/1
  Data Store Read75/1 -> BraSystem/1(BraPre_act_l)
  Data Store Read74/1 -> BraSystem/2(BraPre_act_r)
  Constant2/1 -> Battery/1(pwr_dis_bat)
  Data Store Read50/1 -> Terminator10/1
  Data Store Read54/1 -> Terminator11/1
  Data Store Read55/1 -> Terminator12/1
  Data Store Read56/1 -> Terminator13/1
  Data Store Read62/1 -> Terminator14/1
  Data Store Read65/1 -> Terminator15/1
  Data Store Read52/1 -> Terminator16/1
  Data Store Read53/1 -> Terminator17/1
  Data Store Read38/1 -> Terminator18/1
  Data Store Read42/1 -> Terminator19/1
  Data Store Read43/1 -> Terminator20/1
  Data Store Read44/1 -> Terminator21/1
  Data Store Read45/1 -> Terminator22/1
  Data Store Read48/1 -> Terminator23/1
  Data Store Read40/1 -> Terminator24/1
  Data Store Read41/1 -> Terminator25/1
  Data Store Read18/1 -> Terminator26/1
  Data Store Read22/1 -> Terminator27/1
  Data Store Read23/1 -> Terminator28/1
  Data Store Read24/1 -> Terminator29/1
  Data Store Read25/1 -> Terminator30/1
  Data Store Read29/1 -> Terminator31/1
  Data Store Read20/1 -> Terminator32/1
  Data Store Read21/1 -> Terminator33/1
  Data Store Read14/1 -> Terminator34/1
  Data Store Read26/1 -> Terminator35/1
  Data Store Read31/1 -> Terminator36/1
  Data Store Read32/1 -> Terminator37/1
  Data Store Read33/1 -> Terminator38/1
  Data Store Read36/1 -> Terminator39/1
  Data Store Read16/1 -> Terminator40/1
  Data Store Read17/1 -> Terminator41/1
  Data Store Read67/1 -> Terminator42/1
  Data Store Read68/1 -> Terminator43/1
  Data Store Read69/1 -> Terminator44/1
  Data Store Read70/1 -> Terminator45/1
  Data Store Read71/1 -> Terminator46/1
  Data Store Read72/1 -> Terminator47/1
  Data Store Read73/1 -> Terminator48/1
  Data Type Conversion/1 -> DriveMotor/4(trqlimL_dig_lf)
  Data Type Conversion1/1 -> DriveMotor/9(trqlimL_dig_lr)
  Data Type Conversion2/1 -> DriveMotor/14(trqlimL_dig_rf)
  Data Type Conversion3/1 -> DriveMotor/19(trqlimL_dig_rr)
  MATLAB Function/1(guzhang_lf) -> DriveMotor/5(guzhang_lf)
  MATLAB Function1/1(guzhang_lr) -> DriveMotor/10(guzhang_lr)
  MATLAB Function2/1(guzhang_rf) -> DriveMotor/15(guzhang_rf)
  MATLAB Function3/1(guzhang_rr) -> DriveMotor/20(guzhang_rr)

== system DDCU_wxt_v02_forA_LabviewV02/MainControl ==
  Signals : Inport
  function : TriggerPort  TriggerType=function-call
  Scope : Scope
      settings: TimeRange=20  YMin=4  SaveName=ScopeData53
  SendOutPrepare : Subsystem
  To Workspace : ToWorkspace  VariableName=simout5  SaveFormat=Timeseries  SampleTime=-1
  mode_control : Subsystem
  mode_switch : Subsystem
  wires:
  Signals/1 -> mode_control/2(Signals), mode_switch/1(Signals)
  mode_switch/1(mode_dem_out) -> mode_control/1(mode_dem_out), Scope/1, To Workspace/1
  mode_control/1(com_dem) -> SendOutPrepare/1(com_dem)

== matlab function DDCU_wxt_v02_forA_LabviewV02/MainControl/mode_control/forward/forward/Drive/驱动防滑控制TCS/转向TCS/左转/前后轮均滑转/HeartBeat1 ==
  data: life_pre input; life output
function life = fcn(life_pre)
%#codegen
life=life_pre+1;
if life>15
    life=0;
end
end

== matlab function DDCU_wxt_v02_forA_LabviewV02/MainControl/mode_control/forward/forward/Drive/驱动防滑控制TCS/转向TCS/右转/MATLAB Function2 ==
  data: s_act_rf input; flag_rf output; s_opt_zhuan input; s_opt_zhuan_add input; flag_rf_pre input
function flag_rf = fcn(s_act_rf,s_opt_zhuan,s_opt_zhuan_add,flag_rf_pre)
%#codegen
if s_act_rf>s_opt_zhuan+s_opt_zhuan_add
    flag_rf=1;
elseif s_act_rf<s_opt_zhuan
    flag_rf = 0;
else
    flag_rf=flag_rf_pre;
end
end

== matlab function DDCU_wxt_v02_forA_LabviewV02/MainControl/mode_control/forward/forward/Drive/驱动防滑控制TCS/转向TCS/右转/前轮滑转/HeartBeat ==
  data: life_pre input; life output
function life = fcn(life_pre)
%#codegen
life=life_pre+1;
if life>15
    life=0;
end
end

== matlab function DDCU_wxt_v02_forA_LabviewV02/MainControl/mode_control/forward/forward/Drive/驱动防滑控制TCS/转向TCS/右转/后轮滑转/HeartBeat ==
  data: life_pre input; life output
function life = fcn(life_pre)
%#codegen
life=life_pre+1;
if life>15
    life=0;
end
end

== matlab function DDCU_wxt_v02_forA_LabviewV02/MainControl/mode_control/forward/forward/Drive/驱动防滑控制TCS/转向TCS/右转/前后轮均滑转/HeartBeat1 ==
  data: life_pre input; life output
function life = fcn(life_pre)
%#codegen
life=life_pre+1;
if life>15
    life=0;
end
end

== matlab function DDCU_wxt_v02_forA_LabviewV02/MainControl/mode_control/forward/forward/Brake/MATLAB Function ==
  data: guzhang_lf input; gz_total output; guzhang_lr input; guzhang_rf input; guzhang_rr input
function gz_total = fcn(guzhang_lf,guzhang_lr,guzhang_rf,guzhang_rr)
%#codegen
if guzhang_lf==0 && guzhang_lr==0 && guzhang_rf==0 && guzhang_rr==0
    gz_total=0;
else
    gz_total=1;
end
end

== matlab function DDCU_wxt_v02_forA_LabviewV02/MainControl/mode_control/forward/forward/Brake/MATLAB Function4 ==
  data: syi_act_rr input; flagyi_rr output; s_opt_yi input; s_opt_yi_add input; flagyi_rr_pre input
function flagyi_rr = fcn(syi_act_rr,s_opt_yi,s_opt_yi_add,flagyi_rr_pre)
%#codegen
if syi_act_rr>s_opt_yi+s_opt_yi_add
    flagyi_rr=1;
elseif syi_act_rr<s_opt_yi
    flagyi_rr = 0;
else
    flagyi_rr=flagyi_rr_pre;
end
end

== matlab function DDCU_wxt_v02_forA_LabviewV02/MainControl/mode_control/neutral/neutral/HeartBeat1 ==
  data: life_pre input; life output
function life = fcn(life_pre)
%#codegen
life=life_pre+1;
if life>15
    life=0;
end
end

== matlab function DDCU_wxt_v02_forA_LabviewV02/MainControl/mode_control/center_steer/center_steer/HeartBeat1 ==
  data: life_pre input; life output
function life = fcn(life_pre)
%#codegen
life=life_pre+1;
if life>15
    life=0;
end
end
